simulink model "lab2_task4"  (R2020a)
settings: Solver=FixedStepDiscrete  StartTime=0.0  StopTime=inf  FixedStep=0.02  RelTol=1e-3  EnableMultiTasking=on
values from neighbouring files (symbols this model uses):
  a = 1    [lab2_task3_4_trajectories.m]    (also in plot_lidar.m)
  b = -2    [lab2_task3_4_trajectories.m]
  c = 4    [lab2_task3_4_trajectories.m]
undefined symbols (not defined in the file or in its folder): angdiff, Angular, Linear
libraries: robotlib x3, robotcorelib x1
settings Model: Creator=The MathWorks, Inc.  LastModifiedBy=Pablo
settings DataIOCC: LimitDataPoints=on  SaveFormat=Array  ReturnWorkspaceOutputs=off
settings OptimizationCC: ZeroExternalMemoryAtStartup=off  ZeroInternalMemoryAtStartup=off  LifeSpan=Inf  MaxStackSize=64
settings DebuggingCC: SolverPrmCheckMsg=warning  AllowSymbolicDim=off  SFUnexpectedBacktrackingDiag=warning  SFNoUnconditionalDefaultTransitionDiag=warning  SFExecutionAtInitializationDiag=none  ArithmeticOperatorsInVariantConditions=warning
settings HardwareCC: ProdBitPerPointer=32  ProdBitPerSizeT=32  ProdBitPerPtrDiffT=32  ProdLargestAtomicFloat=None  ProdIntDivRoundTo=Undefined  ProdEndianess=Unspecified  ProdWordSize=32  ProdHWDeviceType=Generic->Unspecified (assume 32-bit Generic)  TargetHWDeviceType=Generic->Unspecified (assume 32-bit Generic)  UseEmbeddedCoderFeatures=off
settings ModelReferenceCC: PropagateSignalLabelsOutOfModel=off
settings SFSimCC: SimUseLocalCustomCode=off  CustomCodeUndefinedFunction=UseInterfaceOnly
settings RTWCC: SystemTargetFile=ert.tlc  HardwareBoard=Robot Operating System (ROS)  TemplateMakefile=ert_default_tmf  RTWUseLocalCustomCode=off  Toolchain=Catkin  TargetLang=C++
settings CodeAppCC: StateflowObjectComments=on
settings ERTTargetCC: MultiwordLength=2048  ERTCustomFileBanners=off  MultiInstanceERTCode=on  CodeInterfacePackaging=C++ class  SupportContinuousTime=on  SupportNonInlinedSFcns=on  RemoveResetFunc=off  SupportVariableSizeSignals=on  ModelStepFunctionPrototypeControlCompliant=off  RootIOFormat=Structure reference  ConvertIfToSwitch=off  SuppressUnreachableDefaultCases=off
settings ConfigComp: CovMetricSettings=dw  CovHtmlReporting=on  CovSaveCumulativeToWorkspaceVar=on  CovSaveSingleToWorkspaceVar=on  CovExternalEMLEnable=off  CovSFcnEnable=off

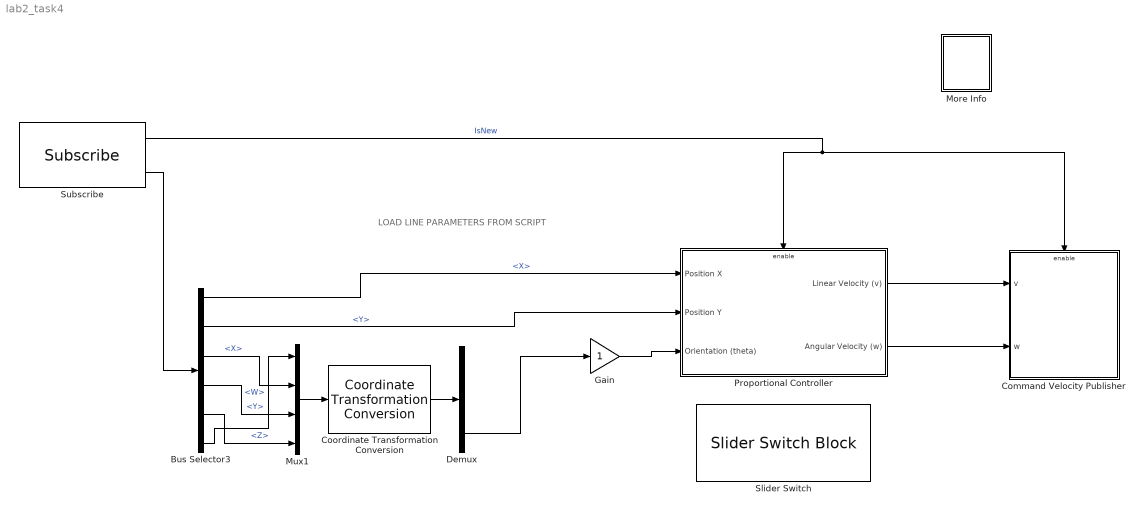
== system lab2_task4 ==
  note: LOAD LINE PARAMETERS FROM SCRIPT
  Bus Selector3 : BusSelector  OutputSignals=Pose.Pose.Position.X,Pose.Pose.Position.Y,Pose.Pose.Orientation.X,Pose.Pose.Orientation.Y,Pose.Pose.Orientation.Z,Pose.Pose.Orientation.W
  Command Velocity Publisher : Subsystem
  Coordinate Transformation Conversion : robotcorelib/Coordinate Transformation Conversion  InputRepresentation=Quaternion  InputEulerSequence=XYZ  ShowTrVecInputPort=on  OutputRepresentation=Euler Angles  OutputEulerSequence=XYZ  ShowTrVecOutputPort=on  SimulateUsing=Interpreted execution
      settings: SourceProductBaseCode=NV,RO,RR
  Demux : Demux  Outputs=3
  Gain : Gain
  More Info : Subsystem
      settings: OpenFcn=showdemo(bdroot(gcb))
      mask Display: disp('?')
  Mux1 : Mux
  Proportional Controller : Subsystem
  Slider Switch : SliderSwitchBlock
      settings: Values={{'STOP OFF', 'STOP ON'}, [0 1]}
  Subscribe : robotlib/Subscribe  topicSource=Select from ROS network  topic=/odom  messageType=nav_msgs/Odometry  sampleTime=-1  messageQueueLength=51
  wires:
  Subscribe/2 -> Bus Selector3/1
  Subscribe/1 -> Proportional Controller/Enable, Command Velocity Publisher/Enable  "IsNew"
  Mux1/1 -> Coordinate Transformation Conversion/1
  Coordinate Transformation Conversion/1 -> Demux/1
  Proportional Controller/2(Angular Velocity (w)) -> Command Velocity Publisher/2(w)
  Proportional Controller/1(Linear Velocity (v)) -> Command Velocity Publisher/1(v)
  Bus Selector3/1 -> Proportional Controller/1(Position X)  "<X>"
  Bus Selector3/2 -> Proportional Controller/2(Position Y)  "<Y>"
  Gain/1 -> Proportional Controller/3(Orientation (theta))
  Bus Selector3/3 -> Mux1/2  "<X>"
  Bus Selector3/4 -> Mux1/3  "<Y>"
  Bus Selector3/5 -> Mux1/4  "<Z>"
  Bus Selector3/6 -> Mux1/1  "<W>"
  Demux/3 -> Gain/1

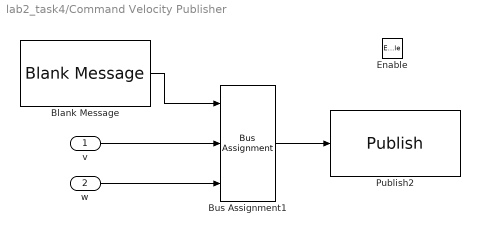
== system lab2_task4/Command Velocity Publisher ==
  v : Inport
  w : Inport  Port=2
  Enable : EnablePort
  Blank Message : robotlib/Blank Message  messageClass=Message  entityType=geometry_msgs/Twist  messageType=geometry_msgs/Twist  SampleTime=inf
  Bus Assignment1 : BusAssignment  DialogController=Simulink.DDGSource_BusAssignment  AssignedSignals=Linear.X,Angular.Z
  Publish2 : robotlib/Publish  topicSource=Select from ROS network  topic=/cmd_vel  messageType=geometry_msgs/Twist  messageQueueLength=105
  wires:
  Bus Assignment1/1 -> Publish2/1
  Blank Message/1 -> Bus Assignment1/1
  v/1 -> Bus Assignment1/2
  w/1 -> Bus Assignment1/3

== system lab2_task4/More Info ==

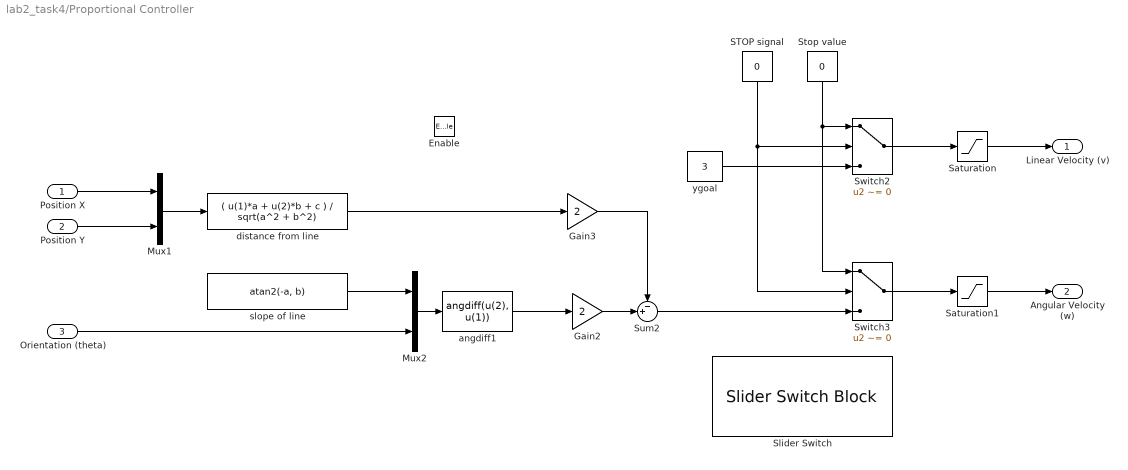
== system lab2_task4/Proportional Controller ==
  Position X : Inport
  Position Y : Inport  Port=2
  Orientation (theta) : Inport  Port=3
  Enable : EnablePort
  Gain2 : Gain  Gain=2
  Gain3 : Gain  Gain=2
  Mux1 : Mux  Inputs=2
  Mux2 : Mux  Inputs=2
  STOP signal : Constant  Value=0
  Saturation : Saturate  UpperLimit=0.3  LinearizeAsGain=off
  Saturation1 : Saturate  LinearizeAsGain=off
  Slider Switch : SliderSwitchBlock
      settings: Values={{'STOP OFF', 'STOP ON'}, [0 1]}
  Stop value : Constant  Value=0
  Sum2 : Sum  Inputs=-+|
  Switch2 : Switch  Criteria=u2 ~= 0
  Switch3 : Switch  Criteria=u2 ~= 0
  angdiff1 : MATLABFcn  MATLABFcn=angdiff(u(2), u(1))  OutputDimensions=1  Output1D=off
  distance from line : MATLABFcn  MATLABFcn=( u(1)*a + u(2)*b + c ) / sqrt(a^2 + b^2)  OutputDimensions=1  Output1D=off
  slope of line : MATLABFcn  MATLABFcn=atan2(-a, b)  OutputDimensions=1  Output1D=off
  ygoal : Constant  Value=3
  Linear Velocity (v) : Outport  VectorParamsAs1DForOutWhenUnconnected=off
  Angular Velocity (w) : Outport  Port=2  VectorParamsAs1DForOutWhenUnconnected=off
  wires:
  Stop value/1 -> Switch2/1, Switch3/1
  Saturation/1 -> Linear Velocity (v)/1
  Switch2/1 -> Saturation/1
  Switch3/1 -> Saturation1/1
  Saturation1/1 -> Angular Velocity (w)/1
  STOP signal/1 -> Switch2/2, Switch3/2
  Position X/1 -> Mux1/1
  Position Y/1 -> Mux1/2
  Mux1/1 -> distance from line/1
  distance from line/1 -> Gain3/1
  Gain2/1 -> Sum2/2
  Gain3/1 -> Sum2/1
  ygoal/1 -> Switch2/3
  Mux2/1 -> angdiff1/1
  Orientation (theta)/1 -> Mux2/2
  angdiff1/1 -> Gain2/1
  Sum2/1 -> Switch3/3
  slope of line/1 -> Mux2/1
